simulink model "a_1b2c1d0"  (Simulink 7.9)
settings: Solver=ode45  StartTime=0.0  StopTime=10.0  RelTol=1e-3
settings Model: Creator=Hugo  LastModifiedBy=Hugo
settings DataIOCC: LimitDataPoints=off

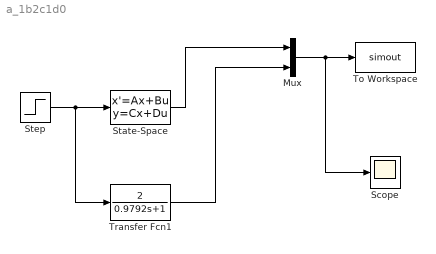
== system a_1b2c1d0 ==
  Mux : Mux  Inputs=2
  Scope : Scope
      settings: SampleInput=on  SampleTime=0.01
  State-Space : StateSpace  A=-1  B=2  D=0
  Step : Step  Time=0  After=2  SampleTime=0
  To Workspace : ToWorkspace  VariableName=simout  SampleTime=-1
  Transfer Fcn1 : TransferFcn  Numerator=[2]  Denominator=[0.9792 1]
  wires:
  Step/1 -> Transfer Fcn1/1, State-Space/1
  Mux/1 -> To Workspace/1, Scope/1
  Transfer Fcn1/1 -> Mux/2
  State-Space/1 -> Mux/1
